simulink library "sadc_library_old"  (R2020b)
settings: Solver=VariableStepAuto  StartTime=0.0  StopTime=10.0  RelTol=1e-3
undefined symbols (not defined in the file): actuators, constants, control, magnitude, orbit, sensors
libraries: vrlib x12
(part 1 of 2)
settings Model: Creator=loren  LastModifiedBy=loren

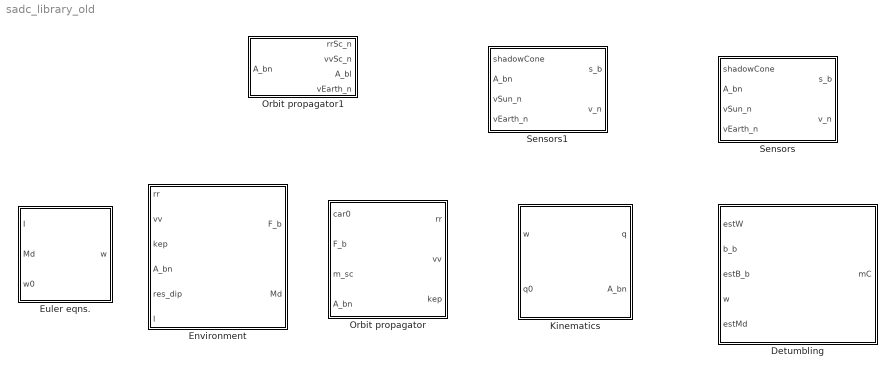
== system sadc_library_old ==
  Detumbling : Subsystem
  Environment : Subsystem
  Euler eqns. : Subsystem
  Kinematics : Subsystem
  Orbit propagator : Subsystem
  Orbit propagator1 : Subsystem
  Sensors : Subsystem
  Sensors1 : Subsystem

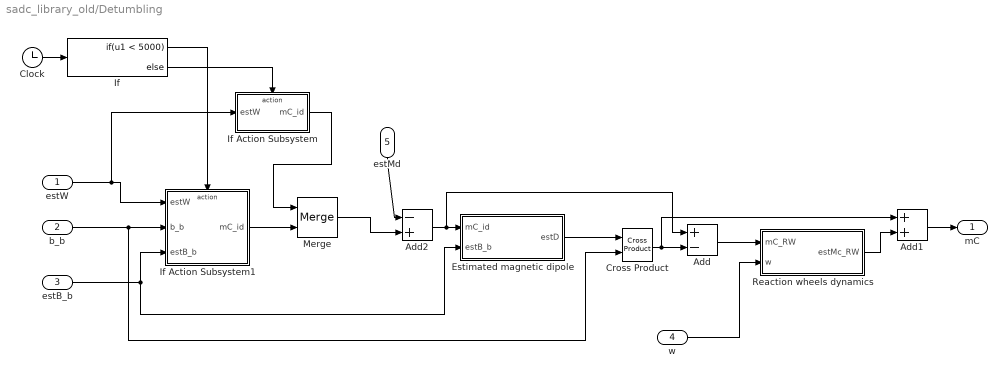
== system sadc_library_old/Detumbling ==
  estW : Inport
  b_b : Inport  Port=2
  estB_b : Inport  Port=3
  w : Inport  Port=4
  estMd : Inport  Port=5
  Add : Sum  Inputs=+-
  Add1 : Sum
  Add2 : Sum  Inputs=-+
  Clock : Clock
  Cross Product : vrlib/Utilities/Cross Product
  Estimated magnetic dipole : Subsystem
  If : If  IfExpression=u1 < 5000
  If Action Subsystem : Subsystem  TreatAsAtomicUnit=on
  If Action Subsystem1 : Subsystem  TreatAsAtomicUnit=on
  Merge : Merge
  Reaction wheels dynamics : Subsystem
  mC : Outport
  wires:
  estW/1 -> If Action Subsystem/1(estW), If Action Subsystem1/1(estW)
  b_b/1 -> If Action Subsystem1/2(b_b), Cross Product/2
  estB_b/1 -> If Action Subsystem1/3(estB_b), Estimated magnetic dipole/2(estB_b)
  If Action Subsystem1/1(mC_id) -> Merge/2
  Estimated magnetic dipole/1(estD) -> Cross Product/1
  Cross Product/1 -> Add1/1, Add/2
  Add/1 -> Reaction wheels dynamics/1(mC_RW)
  w/1 -> Reaction wheels dynamics/2(w)
  Reaction wheels dynamics/1(estMc_RW) -> Add1/2
  Add1/1 -> mC/1
  Add2/1 -> Estimated magnetic dipole/1(mC_id), Add/1
  estMd/1 -> Add2/1
  Clock/1 -> If/1
  Merge/1 -> Add2/2
  If/1 -> If Action Subsystem1/Action
  If/2 -> If Action Subsystem/Action
  If Action Subsystem/1(mC_id) -> Merge/1

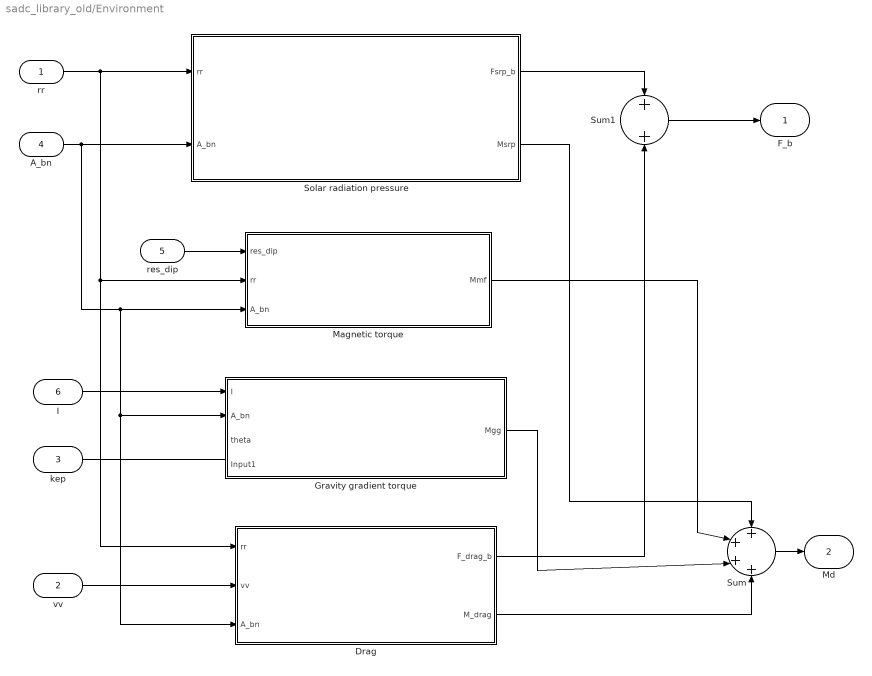
== system sadc_library_old/Environment ==
  rr : Inport
  vv : Inport  Port=2
  kep : Inport  Port=3
  A_bn : Inport  Port=4
  res_dip : Inport  Port=5
  I : Inport  Port=6
  Drag : Subsystem
  Gravity gradient torque : Subsystem
  Magnetic torque : Subsystem
  Solar radiation pressure : Subsystem
  Sum : Sum  Inputs=++++
  Sum1 : Sum
  F_b : Outport
  Md : Outport  Port=2
  wires:
  kep/1 -> ?
  Solar radiation pressure/1(Fsrp_b) -> Sum1/1
  Solar radiation pressure/2(Msrp) -> Sum/1
  A_bn/1 -> Drag/3(A_bn), Gravity gradient torque/2(A_bn), Magnetic torque/3(A_bn), Solar radiation pressure/2(A_bn)
  vv/1 -> Drag/2(vv)
  rr/1 -> Magnetic torque/2(rr), Drag/1(rr), Solar radiation pressure/1(rr)
  Gravity gradient torque/1(Mgg) -> Sum/3
  Drag/2(M_drag) -> Sum/4
  Drag/1(F_drag_b) -> Sum1/2
  I/1 -> Gravity gradient torque/1(I)
  res_dip/1 -> Magnetic torque/1(res_dip)
  Magnetic torque/1(Mmf) -> Sum/2
  Sum1/1 -> F_b/1
  Sum/1 -> Md/1

== system sadc_library_old/Euler eqns. ==
  I : Inport
  Md : Inport  Port=2
  w0 : Inport  Port=3
  Add : Sum  Inputs=-+
  Cross Product : vrlib/Utilities/Cross Product
  Divide : Product  Inputs=/*  Multiplication=Matrix(*)
  Integrator : Integrator  InitialConditionSource=external
  Product : Product  Multiplication=Matrix(*)
  w : Outport
  wires:
  I/1 -> Divide/1, Product/1
  w0/1 -> Integrator/2
  Integrator/1 -> Product/2, w/1, Cross Product/2  "w"
  Product/1 -> Cross Product/1
  Md/1 -> Add/2
  Cross Product/1 -> Add/1
  Add/1 -> Divide/2
  Divide/1 -> Integrator/1

== system sadc_library_old/Kinematics ==
  w : Inport
  q0 : Inport  Port=2
  DCM : Subsystem
  Quaternion integration : Subsystem
  q : Outport
  A_bn : Outport  Port=2
  wires:
  w/1 -> Quaternion integration/1(w)
  q0/1 -> Quaternion integration/2(q0)
  Quaternion integration/1(q) -> q/1, DCM/1(q)
  DCM/1(A_bn) -> A_bn/1

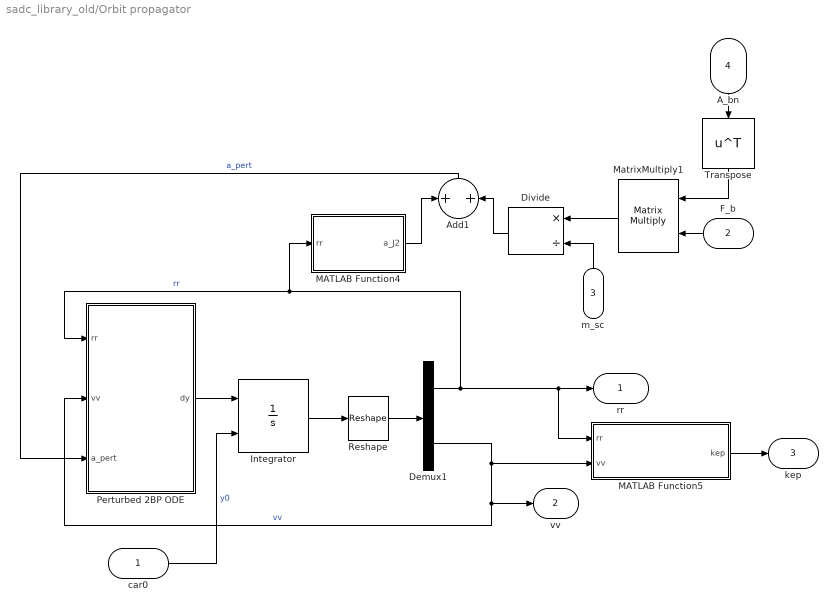
== system sadc_library_old/Orbit propagator ==
  car0 : Inport
  F_b : Inport  Port=2
  m_sc : Inport  Port=3
  A_bn : Inport  Port=4
  Add1 : Sum
  Demux1 : Demux  Outputs=[3,3]
  Divide : Product  Inputs=*/
  Integrator : Integrator  InitialConditionSource=external
  MATLAB Function4 : MATLAB Function  TreatAsAtomicUnit=on
  MATLAB Function5 : MATLAB Function  TreatAsAtomicUnit=on
  MatrixMultiply1 : Product  Multiplication=Matrix(*)
  Perturbed 2BP ODE : Subsystem
  Reshape : Reshape  OutputDimensionality=Column vector (2-D)
  Transpose : Math  Operator=transpose  SaturateOnIntegerOverflow=on
  rr : Outport
  vv : Outport  Port=2
  kep : Outport  Port=3
  wires:
  Integrator/1 -> Reshape/1
  Demux1/1 -> MATLAB Function5/1(rr), rr/1, MATLAB Function4/1(rr), Perturbed 2BP ODE/1(rr)  "rr"
  Perturbed 2BP ODE/1(dy) -> Integrator/1
  Demux1/2 -> vv/1, Perturbed 2BP ODE/2(vv), MATLAB Function5/2(vv)  "vv"
  car0/1 -> Integrator/2  "y0"
  Add1/1 -> Perturbed 2BP ODE/3(a_pert)  "a_pert"
  MATLAB Function4/1(a_J2) -> Add1/1
  F_b/1 -> MatrixMultiply1/2
  MatrixMultiply1/1 -> Divide/1
  m_sc/1 -> Divide/2
  Divide/1 -> Add1/2
  MATLAB Function5/1(kep) -> kep/1
  A_bn/1 -> Transpose/1
  Transpose/1 -> MatrixMultiply1/1
  Reshape/1 -> Demux1/1

== system sadc_library_old/Orbit propagator1 ==
  A_bn : Inport
  Gain : Gain
  Integrator : Integrator  InitialCondition=orbit.theta0
  LVLH frame : Subsystem
  Normalize Vector : vrlib/Utilities/Normalize Vector  maxzero=0
  Position and velocity (inertial frame) : Subsystem
  True anomaly ODE : Subsystem
  rrSc_n : Outport
  vvSc_n : Outport  Port=2
  A_bl : Outport  Port=3
  vEarth_n : Outport  Port=4
  wires:
  Gain/1 -> vEarth_n/1
  Normalize Vector/1 -> Gain/1
  A_bn/1 -> LVLH frame/2(A_bn)
  LVLH frame/1(A_bl) -> A_bl/1
  Position and velocity (inertial frame)/2(vvSc_n) -> vvSc_n/1
  Position and velocity (inertial frame)/1(rrSc_n) -> rrSc_n/1, Normalize Vector/1
  Integrator/1 -> LVLH frame/1(theta), Position and velocity (inertial frame)/1(theta), True anomaly ODE/1(theta)
  True anomaly ODE/1(theta_dot) -> Integrator/1

== system sadc_library_old/Sensors ==
  shadowCone : Inport
  A_bn : Inport  Port=2
  vSun_n : Inport  Port=3
  vEarth_n : Inport  Port=4
  Eclipse (S.T + E.H sensors) : Subsystem  TreatAsAtomicUnit=on
  Merge : Merge
  Merge2 : Merge
  Sunlight (S.S + E.H sensors) : Subsystem  TreatAsAtomicUnit=on
  s_b : Outport
  v_n : Outport  Port=2
  wires:
  shadowCone/1 -> Eclipse (S.T + E.H sensors)/Enable, Sunlight (S.S + E.H sensors)/Enable
  A_bn/1 -> Eclipse (S.T + E.H sensors)/1(A_bn), Sunlight (S.S + E.H sensors)/1(A_bn)
  vSun_n/1 -> Sunlight (S.S + E.H sensors)/2(vSun_n)
  vEarth_n/1 -> Sunlight (S.S + E.H sensors)/3(vEarth_n), Eclipse (S.T + E.H sensors)/2(vEarth_n)
  Merge/1 -> s_b/1
  Merge2/1 -> v_n/1
  Eclipse (S.T + E.H sensors)/1(s_b) -> Merge/1
  Sunlight (S.S + E.H sensors)/1(s_b) -> Merge/2
  Sunlight (S.S + E.H sensors)/2(v_n) -> Merge2/2
  Eclipse (S.T + E.H sensors)/2(v_n) -> Merge2/1

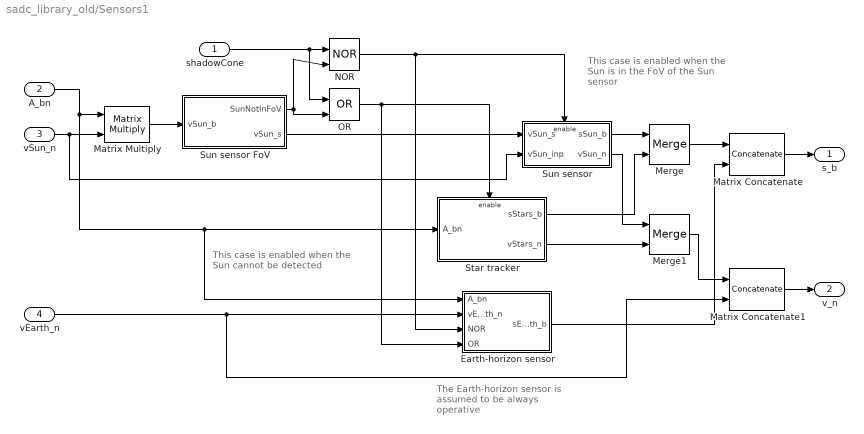
== system sadc_library_old/Sensors1 ==
  note: The Earth-horizon sensor
      | is assumed to be always
      | operative
  note: This case is enabled when
      | the Sun cannot be detected
  note: This case is enabled when
      | the Sun is in the FoV
      | of the Sun sensor
  shadowCone : Inport
  A_bn : Inport  Port=2
  vSun_n : Inport  Port=3
  vEarth_n : Inport  Port=4
  Earth-horizon sensor : Subsystem
  Matrix Concatenate : Concatenate  Mode=Multidimensional array  ConcatenateDimension=2
  Matrix Concatenate1 : Concatenate  Mode=Multidimensional array  ConcatenateDimension=2
  Matrix Multiply : Product  Multiplication=Matrix(*)
  Merge : Merge
  Merge1 : Merge
  NOR : Logic  Operator=NOR  IconShape=distinctive  AllPortsSameDT=off  OutDataTypeStr=boolean
  OR : Logic  Operator=OR  IconShape=distinctive  AllPortsSameDT=off  OutDataTypeStr=boolean
  Star tracker : Subsystem
  Sun sensor : Subsystem
  Sun sensor FoV : Subsystem
  s_b : Outport
  v_n : Outport  Port=2
  wires:
  A_bn/1 -> Earth-horizon sensor/1(A_bn), Star tracker/1(A_bn), Matrix Multiply/1
  vSun_n/1 -> Sun sensor/2(vSun_inp), Matrix Multiply/2
  Matrix Multiply/1 -> Sun sensor FoV/1(vSun_b)
  shadowCone/1 -> NOR/1, OR/1
  Sun sensor FoV/1(SunNotInFoV) -> NOR/2, OR/2
  Sun sensor FoV/2(vSun_s) -> Sun sensor/1(vSun_s)
  OR/1 -> Star tracker/Enable, Earth-horizon sensor/4(OR)
  vEarth_n/1 -> Matrix Concatenate1/2, Earth-horizon sensor/2(vEarth_n)
  Sun sensor/1(sSun_b) -> Merge/1
  Star tracker/1(sStars_b) -> Merge/2
  Star tracker/2(vStars_n) -> Merge1/2
  Matrix Concatenate1/1 -> v_n/1
  Matrix Concatenate/1 -> s_b/1
  Sun sensor/2(vSun_n) -> Merge1/1
  Merge/1 -> Matrix Concatenate/1
  Earth-horizon sensor/1(sEarth_b) -> Matrix Concatenate/2
  Merge1/1 -> Matrix Concatenate1/1
  NOR/1 -> Sun sensor/Enable, Earth-horizon sensor/3(NOR)

== system sadc_library_old/Detumbling/Estimated magnetic dipole ==
  mC_id : Inport
  estB_b : Inport  Port=2
  Cross Product : vrlib/Utilities/Cross Product
  Divide : Product  Inputs=/*
  Dot Product : DotProduct  InputSameDT=on  OutDataTypeStr=Inherit: Inherit via internal rule
  Saturation : Saturate  UpperLimit=actuators.mt.D_max  LowerLimit=actuators.mt.D_min
  estD : Outport
  wires:
  Divide/1 -> Saturation/1
  Dot Product/1 -> Divide/1
  Cross Product/1 -> Divide/2
  estB_b/1 -> Dot Product/1, Dot Product/2, Cross Product/1
  mC_id/1 -> Cross Product/2
  Saturation/1 -> estD/1

== system sadc_library_old/Detumbling/If Action Subsystem ==
  estW : Inport
  Action Port : ActionPort
  Gain : Gain  Gain=-control.detumbling.kp
  mC_id : Outport
  wires:
  estW/1 -> Gain/1
  Gain/1 -> mC_id/1

== system sadc_library_old/Detumbling/If Action Subsystem1 ==
  estW : Inport
  b_b : Inport  Port=2
  estB_b : Inport  Port=3
  Action Port : ActionPort
  Cross Product : vrlib/Utilities/Cross Product
  Cross Product1 : vrlib/Utilities/Cross Product
  Gain : Gain  Gain=-control.detumbling.kb
  mC_id : Outport
  wires:
  Cross Product1/1 -> mC_id/1
  estB_b/1 -> Cross Product/1
  estW/1 -> Cross Product/2
  b_b/1 -> Cross Product1/2
  Gain/1 -> Cross Product1/1
  Cross Product/1 -> Gain/1

== system sadc_library_old/Detumbling/Reaction wheels dynamics ==
  mC_RW : Inport
  w : Inport  Port=2
  Add : Sum
  Add1 : Sum  Inputs=--
  Cross Product : vrlib/Utilities/Cross Product
  Gain : Gain  Gain=actuators.rw.A  Multiplication=Matrix(K*u) (u vector)
  Gain1 : Gain  Gain=-actuators.rw.A_star  Multiplication=Matrix(K*u) (u vector)
  Gain2 : Gain  Gain=actuators.rw.A  Multiplication=Matrix(K*u) (u vector)
  Integrator : Integrator  InitialCondition=[0;0;0;0]
  Saturation : Saturate  UpperLimit=actuators.rw.h_max  LowerLimit=-actuators.rw.h_max
  estMc_RW : Outport
  wires:
  mC_RW/1 -> Add/1
  w/1 -> Cross Product/1
  Gain/1 -> Cross Product/2
  Cross Product/1 -> Add1/1, Add/2
  Gain1/1 -> Integrator/1, Gain2/1  "hr_dot"
  Integrator/1 -> Saturation/1  "h_r"
  Saturation/1 -> Gain/1
  Gain2/1 -> Add1/2
  Add1/1 -> estMc_RW/1
  Add/1 -> Gain1/1

== system sadc_library_old/Environment/Drag ==
  rr : Inport
  vv : Inport  Port=2
  A_bn : Inport  Port=3
  Density @ 400 km : Constant  Value=3.725*1e-12
  MATLAB Function1 : MATLAB Function  TreatAsAtomicUnit=on
  F_drag_b : Outport
  M_drag : Outport  Port=2
  wires:
  rr/1 -> MATLAB Function1/1(rr)
  MATLAB Function1/1(Fdrag_b) -> F_drag_b/1
  MATLAB Function1/2(Mdrag) -> M_drag/1
  vv/1 -> MATLAB Function1/2(vv)
  A_bn/1 -> MATLAB Function1/3(A_bn)
  Density @ 400 km/1 -> MATLAB Function1/4(rho)

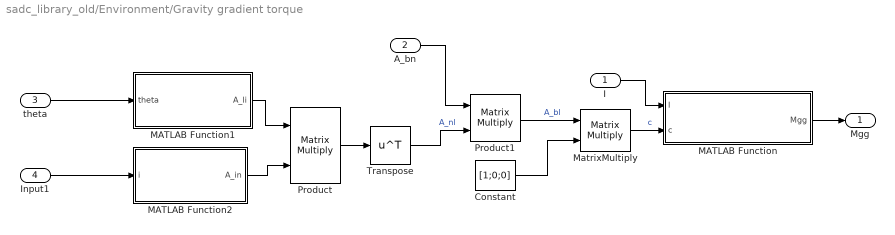
== system sadc_library_old/Environment/Gravity gradient torque ==
  I : Inport
  A_bn : Inport  Port=2
  theta : Inport  Port=3
  Input1 : Inport  Port=4
  Constant : Constant  Value=[1;0;0]
  MATLAB Function : MATLAB Function  TreatAsAtomicUnit=on
  MATLAB Function1 : MATLAB Function  TreatAsAtomicUnit=on
  MATLAB Function2 : MATLAB Function  TreatAsAtomicUnit=on
  MatrixMultiply : Product  Multiplication=Matrix(*)
  Product : Product  Multiplication=Matrix(*)
  Product1 : Product  Multiplication=Matrix(*)
  Transpose : Math  Operator=transpose  SaturateOnIntegerOverflow=on
  Mgg : Outport
  wires:
  I/1 -> MATLAB Function/1(I)
  Product/1 -> Transpose/1
  Transpose/1 -> Product1/2  "A_nl"
  Product1/1 -> MatrixMultiply/1  "A_bl"
  A_bn/1 -> Product1/1
  Constant/1 -> MatrixMultiply/2
  MatrixMultiply/1 -> MATLAB Function/2(c)  "c"
  MATLAB Function/1(Mgg) -> Mgg/1
  MATLAB Function2/1(A_in) -> Product/2
  MATLAB Function1/1(A_li) -> Product/1
  theta/1 -> MATLAB Function1/1(theta)
  Input1/1 -> MATLAB Function2/1(i)

== system sadc_library_old/Environment/Magnetic torque ==
  res_dip : Inport
  rr : Inport  Port=2
  A_bn : Inport  Port=3
  Clock : Clock
  Cross Product : vrlib/Utilities/Cross Product
  MATLAB Function : MATLAB Function  TreatAsAtomicUnit=on
  MATLAB Function1 : MATLAB Function  TreatAsAtomicUnit=on
  Mmf : Outport
  wires:
  Cross Product/1 -> Mmf/1
  Clock/1 -> MATLAB Function1/1(t)
  rr/1 -> MATLAB Function/2(rr)
  A_bn/1 -> MATLAB Function/3(A_bn)
  res_dip/1 -> Cross Product/1
  MATLAB Function/1(b_b) -> Cross Product/2
  MATLAB Function1/1(m) -> MATLAB Function/1(m)

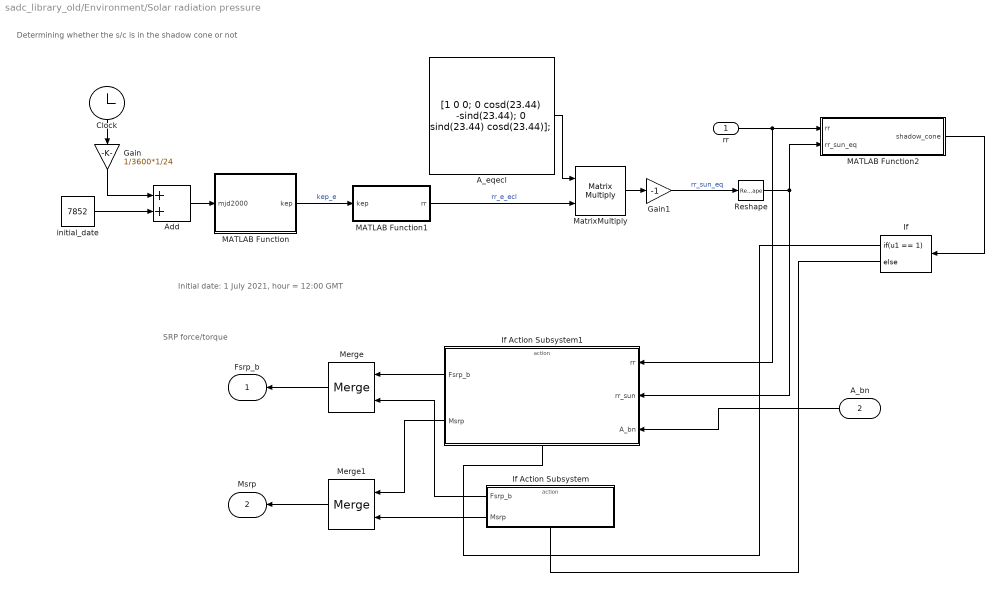
== system sadc_library_old/Environment/Solar radiation pressure ==
  note: SRP force/torque
  note: Initial date: 1 July 2021,
      | hour = 12:00 GMT
  note: Determining whether the s/c is in the shadow cone or not
  rr : Inport
  A_bn : Inport  Port=2
  A_eqecl : Constant  Value=|
      | [1   0   0;
      |     0  cosd(23.44)  -sind(23.44);
      |     0  sind(23.44)  cosd(23.44)];
  Add : Sum
  Clock : Clock
  Gain : Gain  Gain=1/3600*1/24
  Gain1 : Gain  Gain=-1
  If : If  IfExpression=u1 == 1
  If Action Subsystem : Subsystem  TreatAsAtomicUnit=on
  If Action Subsystem1 : Subsystem  TreatAsAtomicUnit=on
  MATLAB Function : MATLAB Function  TreatAsAtomicUnit=on
  MATLAB Function1 : MATLAB Function  TreatAsAtomicUnit=on
  MATLAB Function2 : MATLAB Function  TreatAsAtomicUnit=on
  MatrixMultiply : Product  Multiplication=Matrix(*)
  Merge : Merge
  Merge1 : Merge
  Reshape : Reshape  OutputDimensionality=Column vector (2-D)
  initial_date : Constant  Value=7852
  Fsrp_b : Outport
  Msrp : Outport  Port=2
  wires:
  initial_date/1 -> Add/2
  Clock/1 -> Gain/1
  Add/1 -> MATLAB Function/1(mjd2000)
  Gain/1 -> Add/1
  MatrixMultiply/1 -> Gain1/1
  MATLAB Function1/1(rr) -> MatrixMultiply/2  "rr_e_ecl"
  MATLAB Function/1(kep) -> MATLAB Function1/1(kep)  "kep_e"
  Gain1/1 -> Reshape/1  "rr_sun_eq"
  MATLAB Function2/1(shadow_cone) -> If/1
  If/2 -> If Action Subsystem/Action
  If/1 -> If Action Subsystem1/Action
  If Action Subsystem/1(Fsrp_b) -> Merge/2
  If Action Subsystem/2(Msrp) -> Merge1/2
  rr/1 -> MATLAB Function2/1(rr), If Action Subsystem1/1(rr)
  Merge/1 -> Fsrp_b/1
  Merge1/1 -> Msrp/1
  If Action Subsystem1/1(Fsrp_b) -> Merge/1
  If Action Subsystem1/2(Msrp) -> Merge1/1
  A_bn/1 -> If Action Subsystem1/3(A_bn)
  A_eqecl/1 -> MatrixMultiply/1
  Reshape/1 -> MATLAB Function2/2(rr_sun_eq), If Action Subsystem1/2(rr_sun)

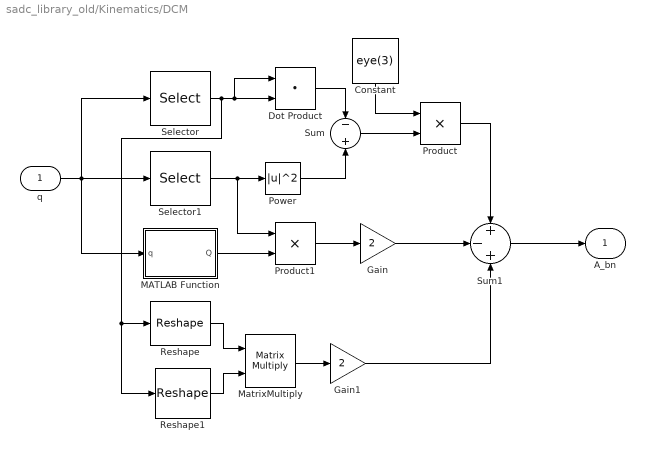
== system sadc_library_old/Kinematics/DCM ==
  q : Inport
  Constant : Constant  Value=eye(3)
  Dot Product : DotProduct  InputSameDT=on  OutDataTypeStr=Inherit: Inherit via internal rule
  Gain : Gain  Gain=2
  Gain1 : Gain  Gain=2
  MATLAB Function : MATLAB Function  TreatAsAtomicUnit=on
  MatrixMultiply : Product  Multiplication=Matrix(*)
  Power : Math  Operator=magnitude^2  SaturateOnIntegerOverflow=on
  Product : Product
  Product1 : Product
  Reshape : Reshape  OutputDimensionality=Column vector (2-D)
  Reshape1 : Reshape  OutputDimensionality=Row vector (2-D)
  Selector : Selector  InputPortWidth=4  IndexOptions=Index vector (dialog)  Indices=[1 2 3]  OutputSizes=1
  Selector1 : Selector  InputPortWidth=4  IndexOptions=Index vector (dialog)  Indices=[4]  OutputSizes=1
  Sum : Sum  Inputs=-+
  Sum1 : Sum  Inputs=+-+
  A_bn : Outport
  wires:
  q/1 -> MATLAB Function/1(q), Selector1/1, Selector/1
  Selector/1 -> Reshape1/1, Reshape/1, Dot Product/2, Dot Product/1
  Selector1/1 -> Product1/1, Power/1
  Power/1 -> Sum/2
  Dot Product/1 -> Sum/1
  Constant/1 -> Product/1
  Sum/1 -> Product/2
  MATLAB Function/1(Q) -> Product1/2
  Product1/1 -> Gain/1
  Reshape/1 -> MatrixMultiply/1
  Reshape1/1 -> MatrixMultiply/2
  MatrixMultiply/1 -> Gain1/1
  Product/1 -> Sum1/1
  Gain/1 -> Sum1/2
  Gain1/1 -> Sum1/3
  Sum1/1 -> A_bn/1

== system sadc_library_old/Kinematics/Quaternion integration ==
  w : Inport
  q0 : Inport  Port=2
  Gain : Gain  Gain=1/2
  Integrator : Integrator  InitialConditionSource=external
  MATLAB Function : MATLAB Function  TreatAsAtomicUnit=on
  MatrixMultiply : Product  Multiplication=Matrix(*)
  Normalize Vector : vrlib/Utilities/Normalize Vector  maxzero=0
  q : Outport
  wires:
  Integrator/1 -> Normalize Vector/1
  w/1 -> MATLAB Function/1(w)
  Normalize Vector/1 -> q/1, MatrixMultiply/2
  q0/1 -> Integrator/2
  MATLAB Function/1(OM_mat) -> MatrixMultiply/1
  MatrixMultiply/1 -> Gain/1
  Gain/1 -> Integrator/1

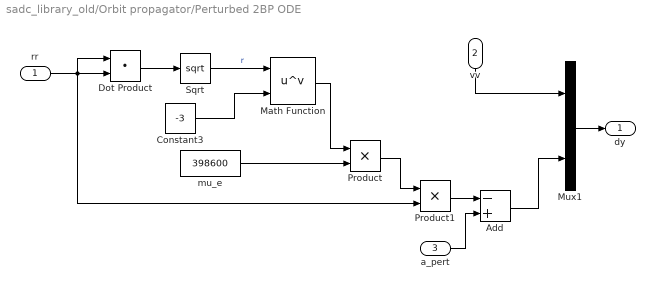
== system sadc_library_old/Orbit propagator/Perturbed 2BP ODE ==
  rr : Inport
  vv : Inport  Port=2
  a_pert : Inport  Port=3
  Add : Sum  Inputs=-+
  Constant3 : Constant  Value=-3
  Dot Product : DotProduct  InputSameDT=on  OutDataTypeStr=Inherit: Inherit via internal rule
  Math Function : Math  Operator=pow  SaturateOnIntegerOverflow=on
  Mux1 : Mux  Inputs=[3,3]
  Product : Product
  Product1 : Product
  Sqrt : Sqrt  SaturateOnIntegerOverflow=on
  mu_e : Constant  Value=398600
  dy : Outport
  wires:
  rr/1 -> Dot Product/1, Product1/2, Dot Product/2
  Add/1 -> Mux1/2
  Math Function/1 -> Product/1
  Mux1/1 -> dy/1
  Dot Product/1 -> Sqrt/1
  Product1/1 -> Add/1
  Product/1 -> Product1/1
  Constant3/1 -> Math Function/2
  a_pert/1 -> Add/2
  Sqrt/1 -> Math Function/1  "r"
  vv/1 -> Mux1/1
  mu_e/1 -> Product/2

== system sadc_library_old/Orbit propagator1/LVLH frame ==
  theta : Inport
  A_bn : Inport  Port=2
  LVLH to inclined orbit frame : Subsystem
  Product : Product  Multiplication=Matrix(*)
  Product1 : Product  Multiplication=Matrix(*)
  R1(i) : Constant  Value=[1 0 0; 0 cos(orbit.i) sin(orbit.i); 0 -sin(orbit.i) cos(orbit.i)];
  Transpose : Math  Operator=transpose  SaturateOnIntegerOverflow=on
  A_bl : Outport
  wires:
  LVLH to inclined orbit frame/1(A_li) -> Product/1
  theta/1 -> LVLH to inclined orbit frame/1(theta)
  R1(i)/1 -> Product/2
  Product1/1 -> A_bl/1  "A_bl"
  A_bn/1 -> Product1/1
  Product/1 -> Transpose/1
  Transpose/1 -> Product1/2  "A_nl"

== system sadc_library_old/Orbit propagator1/Position and velocity (inertial frame) ==
  theta : Inport
  MatrixMultiply : Product  Multiplication=Matrix(*)
  MatrixMultiply1 : Product  Multiplication=Matrix(*)
  Position and velocity (perifocal frame) : Subsystem
  R1(i) : Constant  Value=[1 0 0; 0 cos(orbit.i) sin(orbit.i); 0 -sin(orbit.i) cos(orbit.i)];
  R3(OM) : Constant  Value=[cos(orbit.OM), sin(orbit.OM), 0; -sin(orbit.OM), cos(orbit.OM), 0; 0, 0, 1]
  R3(om) : Constant  Value=[cos(orbit.om), sin(orbit.om), 0; -sin(orbit.om), cos(orbit.om), 0; 0, 0, 1]
  Rotation matrix (perifocal-inertial) : Product  Inputs=3  Multiplication=Matrix(*)
  Transpose : Math  Operator=transpose  SaturateOnIntegerOverflow=on
  rrSc_n : Outport
  vvSc_n : Outport  Port=2
  wires:
  theta/1 -> Position and velocity (perifocal frame)/1(theta)
  Position and velocity (perifocal frame)/1(rrSc_pf) -> MatrixMultiply/2
  R3(OM)/1 -> Rotation matrix (perifocal-inertial)/3
  Transpose/1 -> MatrixMultiply/1, MatrixMultiply1/1
  Rotation matrix (perifocal-inertial)/1 -> Transpose/1
  R1(i)/1 -> Rotation matrix (perifocal-inertial)/2
  R3(om)/1 -> Rotation matrix (perifocal-inertial)/1
  MatrixMultiply1/1 -> vvSc_n/1
  Position and velocity (perifocal frame)/2(vvSc_pf) -> MatrixMultiply1/2
  MatrixMultiply/1 -> rrSc_n/1

== system sadc_library_old/Orbit propagator1/True anomaly ODE ==
  theta : Inport
  Add : Sum
  Constant1 : Constant
  Cos : Trigonometry  Operator=cos
  Gain : Gain  Gain=sqrt(constants.mu/orbit.a^3)
  Gain1 : Gain  Gain=(1 - orbit.e^2)^(-3/2)
  Gain2 : Gain  Gain=orbit.e
  Power : Math  Operator=square  SaturateOnIntegerOverflow=on
  theta_dot : Outport
  wires:
  Gain1/1 -> theta_dot/1
  Gain/1 -> Gain1/1
  Power/1 -> Gain/1
  Add/1 -> Power/1
  Gain2/1 -> Add/2
  Cos/1 -> Gain2/1
  Constant1/1 -> Add/1
  theta/1 -> Cos/1

== system sadc_library_old/Sensors/Eclipse (S.T + E.H sensors) ==
  A_bn : Inport
  vEarth_n : Inport  Port=2
  Enable : EnablePort
  Earth-horizon sensor : Subsystem  AncestorBlock=|
      | library/Sensors/Sunlight
      | (S.S + E.H sensors)/Earth-horizon sensor
  Star tracker : Subsystem
  Vector Concatenate : Concatenate  Mode=Multidimensional array  ConcatenateDimension=2
  Vector Concatenate1 : Concatenate  Mode=Multidimensional array  ConcatenateDimension=2
  s_b : Outport
  v_n : Outport  Port=2
  wires:
  Vector Concatenate1/1 -> v_n/1
  Vector Concatenate/1 -> s_b/1
  Earth-horizon sensor/1(vEarth_b) -> Vector Concatenate/1
  A_bn/1 -> Star tracker/1(A_bn), Earth-horizon sensor/1(A_bn)
  vEarth_n/1 -> Vector Concatenate1/1, Earth-horizon sensor/2(vEarth_n)
  Star tracker/1(sStars_b) -> Vector Concatenate/2
  Star tracker/2(vStars_n) -> Vector Concatenate1/2

== system sadc_library_old/Sensors/Sunlight (S.S + E.H sensors) ==
  A_bn : Inport
  vSun_n : Inport  Port=2
  vEarth_n : Inport  Port=3
  Enable : EnablePort
  Earth-horizon sensor : Subsystem
  Sun sensor : Subsystem
  Vector Concatenate : Concatenate  Mode=Multidimensional array  ConcatenateDimension=2
  Vector Concatenate1 : Concatenate  Mode=Multidimensional array  ConcatenateDimension=2
  s_b : Outport
  v_n : Outport  Port=2
  wires:
  A_bn/1 -> Sun sensor/1(A_bn), Earth-horizon sensor/1(A_bn)
  vSun_n/1 -> Sun sensor/2(vSun_n), Vector Concatenate1/1
  vEarth_n/1 -> Vector Concatenate1/2, Earth-horizon sensor/2(vEarth_n)
  Sun sensor/1(vSun_b) -> Vector Concatenate/1
  Earth-horizon sensor/1(vEarth_b) -> Vector Concatenate/2
  Vector Concatenate/1 -> s_b/1
  Vector Concatenate1/1 -> v_n/1

== system sadc_library_old/Sensors1/Earth-horizon sensor ==
  A_bn : Inport
  vEarth_n : Inport  Port=2
  NOR : Inport  Port=3
  OR : Inport  Port=4
  Constant : Constant  Value=sensors.eh.A_sb
  Determination of the sampling time : Subsystem
  MATLAB Function : MATLAB Function  TreatAsAtomicUnit=on
  MatrixMultiply : Product  Multiplication=Matrix(*)
  MatrixMultiply1 : Product  Multiplication=Matrix(*)
  MatrixMultiply2 : Product  Multiplication=Matrix(*)
  Zero-Order Hold : ZeroOrderHold  SampleTime=max([sensors.ss.Ts, sensors.eh.Ts])
  sEarth_b : Outport
  wires:
  Zero-Order Hold/1 -> MatrixMultiply1/2
  vEarth_n/1 -> MatrixMultiply2/2
  MATLAB Function/1(A_err) -> MatrixMultiply1/1
  A_bn/1 -> MatrixMultiply2/1
  MatrixMultiply1/1 -> sEarth_b/1
  MatrixMultiply/1 -> Zero-Order Hold/1  "vEarth_s"
  MatrixMultiply2/1 -> MatrixMultiply/2
  Constant/1 -> MatrixMultiply/1
  Determination of the sampling time/1(phi) -> MATLAB Function/1(phi)
  Determination of the sampling time/2(theta) -> MATLAB Function/2(theta)
  Determination of the sampling time/3(psi) -> MATLAB Function/3(psi)
  NOR/1 -> Determination of the sampling time/1(NOR)
  OR/1 -> Determination of the sampling time/2(OR)

== system sadc_library_old/Sensors1/Star tracker ==
  A_bn : Inport
  Enable : EnablePort
  MATLAB Function : MATLAB Function  TreatAsAtomicUnit=on
  Memory : Memory  InitialCondition=sensors.st.vStars_n_init  InheritSampleTime=on
  Random Number : RandomNumber  Variance=sensors.st.sigmaPhi^2  Seed=randi(1e5,1,1)  SampleTime=max([sensors.eh.Ts, sensors.st.Ts])
  Random Number1 : RandomNumber  Variance=sensors.st.sigmaTheta^2  Seed=randi(1e5,1,1)  SampleTime=max([sensors.eh.Ts, sensors.st.Ts])
  Random Number2 : RandomNumber  Variance=sensors.st.sigmaPsi^2  Seed=randi(1e5,1,1)  SampleTime=max([sensors.eh.Ts, sensors.st.Ts])
  Reshape : Reshape  OutputDimensionality=Customize  OutputDimensions=[sensors.st.nStars*3, 1]
  Reshape1 : Reshape  OutputDimensionality=Customize  OutputDimensions=[sensors.st.nStars*3, 1]
  Zero-Order Hold : ZeroOrderHold  SampleTime=max([sensors.eh.Ts, sensors.st.Ts])
  sStars_b : Outport
  vStars_n : Outport  Port=2
  wires:
  Memory/1 -> MATLAB Function/5(v_n_old)
  MATLAB Function/2(v_n) -> Reshape1/1, Memory/1
  MATLAB Function/1(s_b) -> Reshape/1
  Zero-Order Hold/1 -> MATLAB Function/1(A_bn)
  Random Number/1 -> MATLAB Function/2(phi)
  Random Number2/1 -> MATLAB Function/4(psi)
  A_bn/1 -> Zero-Order Hold/1
  Random Number1/1 -> MATLAB Function/3(theta)
  Reshape/1 -> sStars_b/1
  Reshape1/1 -> vStars_n/1

== system sadc_library_old/Sensors1/Sun sensor ==
  vSun_s : Inport
  vSun_inp : Inport  Port=2
  Enable : EnablePort
  MATLAB Function : MATLAB Function  TreatAsAtomicUnit=on
  MatrixMultiply1 : Product  Multiplication=Matrix(*)
  Random Number : RandomNumber  Variance=sensors.ss.sigmaPhi^2  Seed=randi(1e5, 1, 1)  SampleTime=max([sensors.ss.Ts, sensors.eh.Ts])
  Random Number1 : RandomNumber  Variance=sensors.ss.sigmaTheta^2  Seed=randi(1e5, 1, 1)  SampleTime=max([sensors.ss.Ts, sensors.eh.Ts])
  Random Number2 : RandomNumber  Variance=sensors.ss.sigmaPsi^2  Seed=randi(1e5, 1, 1)  SampleTime=max([sensors.ss.Ts, sensors.eh.Ts])
  Zero-Order Hold : ZeroOrderHold  SampleTime=max([sensors.ss.Ts, sensors.eh.Ts])
  sSun_b : Outport
  vSun_n : Outport  Port=2
  wires:
  Zero-Order Hold/1 -> MatrixMultiply1/2
  vSun_s/1 -> Zero-Order Hold/1  "vSun_s"
  Random Number2/1 -> MATLAB Function/3(psi)
  MatrixMultiply1/1 -> sSun_b/1
  MATLAB Function/1(A_err) -> MatrixMultiply1/1
  Random Number1/1 -> MATLAB Function/2(theta)
  Random Number/1 -> MATLAB Function/1(phi)
  vSun_inp/1 -> vSun_n/1

== system sadc_library_old/Sensors1/Sun sensor FoV ==
  vSun_b : Inport
  Acos : Trigonometry  Operator=acos
  Constant : Constant  Value=sensors.ss.FoV/2
  Constant1 : Constant  Value=sensors.ss.A_sb
  Dot Product : DotProduct  InputSameDT=on  OutDataTypeStr=Inherit: Inherit via internal rule
  Gain : Gain  Gain=sensors.ss.A_sb  Multiplication=Matrix(K*u) (u vector)
  Less Than : RelationalOperator  Operator=>  OutDataTypeStr=boolean  RndMeth=Simplest
  Normalize Vector : vrlib/Utilities/Normalize Vector  maxzero=0
  Selector : Selector  NumberOfDimensions=2  InputPortWidth=3  IndexOptions=Index vector (dialog),Index vector (dialog)  Indices=[1 2 3],[1]  OutputSizes=1,1
  SunNotInFoV : Outport
  vSun_s : Outport  Port=2
  wires:
  Gain/1 -> vSun_s/1, Dot Product/2
  Selector/1 -> Normalize Vector/1
  Normalize Vector/1 -> Dot Product/1
  vSun_b/1 -> Gain/1
  Dot Product/1 -> Acos/1
  Acos/1 -> Less Than/1
  Constant/1 -> Less Than/2
  Less Than/1 -> SunNotInFoV/1
  Constant1/1 -> Selector/1

== system sadc_library_old/Environment/Solar radiation pressure/If Action Subsystem ==
  Action Port : ActionPort
  Constant : Constant  Value=[0;0;0]
  Constant1 : Constant  Value=[0;0;0]
  Fsrp_b : Outport
  Msrp : Outport  Port=2
  wires:
  Constant/1 -> Fsrp_b/1
  Constant1/1 -> Msrp/1

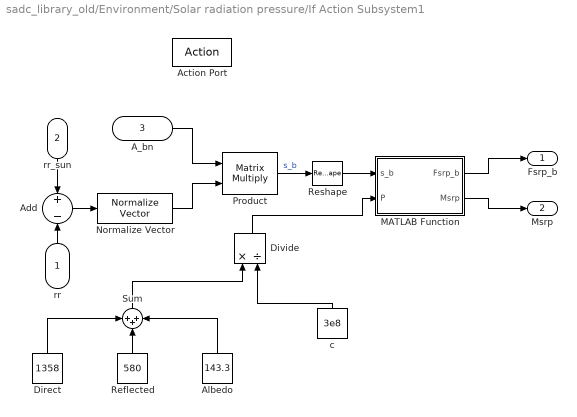
== system sadc_library_old/Environment/Solar radiation pressure/If Action Subsystem1 ==
  rr : Inport
  rr_sun : Inport  Port=2
  A_bn : Inport  Port=3
  Action Port : ActionPort
  Add : Sum  Inputs=+-
  Albedo : Constant  Value=143.3
  Direct : Constant  Value=1358
  Divide : Product  Inputs=*/
  MATLAB Function : MATLAB Function  TreatAsAtomicUnit=on
  Normalize Vector : vrlib/Utilities/Normalize Vector  maxzero=0
  Product : Product  Multiplication=Matrix(*)
  Reflected : Constant  Value=580
  Reshape : Reshape  OutputDimensionality=Column vector (2-D)
  Sum : Sum  Inputs=+++
  c : Constant  Value=3e8
  Fsrp_b : Outport
  Msrp : Outport  Port=2
  wires:
  A_bn/1 -> Product/1
  rr_sun/1 -> Add/1
  Product/1 -> Reshape/1  "s_b"
  Normalize Vector/1 -> Product/2
  Add/1 -> Normalize Vector/1
  MATLAB Function/1(Fsrp_b) -> Fsrp_b/1
  MATLAB Function/2(Msrp) -> Msrp/1
  Reflected/1 -> Sum/2
  Albedo/1 -> Sum/3
  Direct/1 -> Sum/1
  Sum/1 -> Divide/1
  c/1 -> Divide/2
  Divide/1 -> MATLAB Function/2(P)
  rr/1 -> Add/2
  Reshape/1 -> MATLAB Function/1(s_b)

== system sadc_library_old/Orbit propagator1/LVLH frame/LVLH to inclined orbit frame ==
  theta : Inport
  Constant : Constant  Value=0
  Constant1 : Constant  Value=[0 0 1]
  Cos : Trigonometry  Operator=cos
  Gain : Gain  Gain=-1
  Mux : Mux  Inputs=3
  Mux1 : Mux  Inputs=3
  Sin : Trigonometry
  Vector Concatenate : Concatenate  NumInputs=3  Mode=Multidimensional array  ConcatenateDimension=2
  A_li : Outport
  wires:
  Vector Concatenate/1 -> A_li/1
  Mux1/1 -> Vector Concatenate/2
  Constant1/1 -> Vector Concatenate/3
  Mux/1 -> Vector Concatenate/1
  Gain/1 -> Mux1/1
  Constant/1 -> Mux/3, Mux1/3
  Sin/1 -> Mux/2, Gain/1
  Cos/1 -> Mux/1, Mux1/2
  theta/1 -> Cos/1, Sin/1

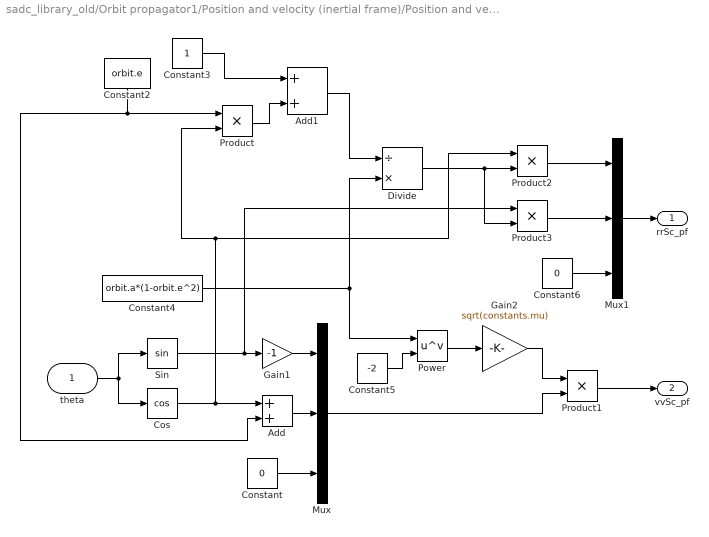
== system sadc_library_old/Orbit propagator1/Position and velocity (inertial frame)/Position and velocity (perifocal frame) ==
  theta : Inport
  Add : Sum
  Add1 : Sum
  Constant : Constant  Value=0
  Constant2 : Constant  Value=orbit.e
  Constant3 : Constant
  Constant4 : Constant  Value=orbit.a*(1-orbit.e^2)
  Constant5 : Constant  Value=-2
  Constant6 : Constant  Value=0
  Cos : Trigonometry  Operator=cos
  Divide : Product  Inputs=/*
  Gain1 : Gain  Gain=-1
  Gain2 : Gain  Gain=sqrt(constants.mu)
  Mux : Mux  Inputs=3
  Mux1 : Mux  Inputs=3
  Power : Math  Operator=pow  SaturateOnIntegerOverflow=on
  Product{,1..3} (4 alike) : Product
  Sin : Trigonometry
  rrSc_pf : Outport
  vvSc_pf : Outport  Port=2
  wires:
  Mux1/1 -> rrSc_pf/1
  Constant6/1 -> Mux1/3
  Product3/1 -> Mux1/2
  Product2/1 -> Mux1/1
  Divide/1 -> Product2/2, Product3/2
  Gain2/1 -> Product1/1
  Power/1 -> Gain2/1
  Constant5/1 -> Power/2
  Constant4/1 -> Power/1, Divide/2
  Add1/1 -> Divide/1
  Product/1 -> Add1/2
  Constant2/1 -> Product/1, Add/2
  Constant3/1 -> Add1/1
  Product1/1 -> vvSc_pf/1
  Constant/1 -> Mux/3
  Add/1 -> Mux/2
  Gain1/1 -> Mux/1
  Cos/1 -> Add/1, Product/2, Product2/1
  Sin/1 -> Gain1/1, Product3/1
  Mux/1 -> Product1/2
  theta/1 -> Sin/1, Cos/1

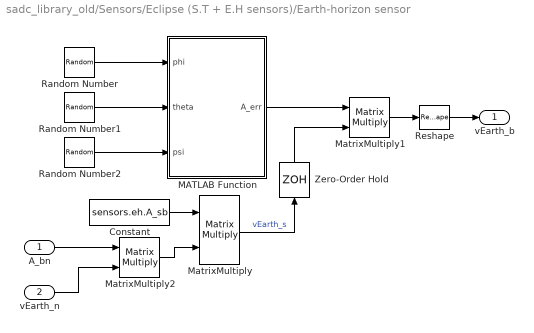
== system sadc_library_old/Sensors/Eclipse (S.T + E.H sensors)/Earth-horizon sensor ==
  A_bn : Inport
  vEarth_n : Inport  Port=2
  Constant : Constant  Value=sensors.eh.A_sb
  MATLAB Function : MATLAB Function  TreatAsAtomicUnit=on
  MatrixMultiply : Product  Multiplication=Matrix(*)
  MatrixMultiply1 : Product  Multiplication=Matrix(*)
  MatrixMultiply2 : Product  Multiplication=Matrix(*)
  Random Number : RandomNumber  Variance=sensors.eh.sigmaPhi^2  Seed=randi(1e5, 1, 1)  SampleTime=max([sensors.eh.Ts, sensors.st.Ts])
  Random Number1 : RandomNumber  Variance=sensors.eh.sigmaTheta^2  Seed=randi(1e5, 1, 1)  SampleTime=max([sensors.eh.Ts, sensors.st.Ts])
  Random Number2 : RandomNumber  Variance=sensors.eh.sigmaPsi^2  Seed=randi(1e5, 1, 1)  SampleTime=max([sensors.eh.Ts, sensors.st.Ts])
  Reshape : Reshape  OutputDimensionality=Column vector (2-D)
  Zero-Order Hold : ZeroOrderHold  SampleTime=max([sensors.eh.Ts, sensors.st.Ts])
  vEarth_b : Outport
  wires:
  Zero-Order Hold/1 -> MatrixMultiply1/2
  vEarth_n/1 -> MatrixMultiply2/2
  MATLAB Function/1(A_err) -> MatrixMultiply1/1
  Random Number2/1 -> MATLAB Function/3(psi)
  A_bn/1 -> MatrixMultiply2/1
  Random Number/1 -> MATLAB Function/1(phi)
  MatrixMultiply1/1 -> Reshape/1
  MatrixMultiply/1 -> Zero-Order Hold/1  "vEarth_s"
  Random Number1/1 -> MATLAB Function/2(theta)
  MatrixMultiply2/1 -> MatrixMultiply/2
  Constant/1 -> MatrixMultiply/1
  Reshape/1 -> vEarth_b/1

== system sadc_library_old/Sensors/Eclipse (S.T + E.H sensors)/Star tracker ==
  A_bn : Inport
  MATLAB Function : MATLAB Function  TreatAsAtomicUnit=on
  Memory : Memory  InitialCondition=sensors.st.vStars_n_init  InheritSampleTime=on
  Random Number : RandomNumber  Variance=sensors.st.sigmaPhi^2  Seed=randi(1e5,1,1)  SampleTime=max([sensors.eh.Ts, sensors.st.Ts])
  Random Number1 : RandomNumber  Variance=sensors.st.sigmaTheta^2  Seed=randi(1e5,1,1)  SampleTime=max([sensors.eh.Ts, sensors.st.Ts])
  Random Number2 : RandomNumber  Variance=sensors.st.sigmaPsi^2  Seed=randi(1e5,1,1)  SampleTime=max([sensors.eh.Ts, sensors.st.Ts])
  Zero-Order Hold : ZeroOrderHold  SampleTime=max([sensors.eh.Ts, sensors.st.Ts])
  sStars_b : Outport
  vStars_n : Outport  Port=2
  wires:
  Random Number1/1 -> MATLAB Function/3(theta)
  A_bn/1 -> Zero-Order Hold/1
  Random Number2/1 -> MATLAB Function/4(psi)
  Random Number/1 -> MATLAB Function/2(phi)
  Zero-Order Hold/1 -> MATLAB Function/1(A_bn)
  MATLAB Function/1(s_b) -> sStars_b/1
  MATLAB Function/2(v_n) -> Memory/1, vStars_n/1
  Memory/1 -> MATLAB Function/5(v_n_old)

== system sadc_library_old/Sensors/Sunlight (S.S + E.H sensors)/Earth-horizon sensor ==
  A_bn : Inport
  vEarth_n : Inport  Port=2
  Constant : Constant  Value=sensors.eh.A_sb
  MATLAB Function : MATLAB Function  TreatAsAtomicUnit=on
  MatrixMultiply : Product  Multiplication=Matrix(*)
  MatrixMultiply1 : Product  Multiplication=Matrix(*)
  MatrixMultiply2 : Product  Multiplication=Matrix(*)
  Random Number : RandomNumber  Variance=sensors.eh.sigmaPhi^2  Seed=randi(1e5, 1, 1)  SampleTime=max([sensors.ss.Ts, sensors.eh.Ts])
  Random Number1 : RandomNumber  Variance=sensors.eh.sigmaTheta^2  Seed=randi(1e5, 1, 1)  SampleTime=max([sensors.ss.Ts, sensors.eh.Ts])
  Random Number2 : RandomNumber  Variance=sensors.eh.sigmaPsi^2  Seed=randi(1e5, 1, 1)  SampleTime=max([sensors.ss.Ts, sensors.eh.Ts])
  Zero-Order Hold : ZeroOrderHold  SampleTime=max([sensors.ss.Ts, sensors.eh.Ts])
  vEarth_b : Outport
  wires:
  Constant/1 -> MatrixMultiply/1
  MatrixMultiply2/1 -> MatrixMultiply/2
  Random Number1/1 -> MATLAB Function/2(theta)
  MatrixMultiply/1 -> Zero-Order Hold/1  "vEarth_s"
  MatrixMultiply1/1 -> vEarth_b/1
  Random Number/1 -> MATLAB Function/1(phi)
  A_bn/1 -> MatrixMultiply2/1
  Random Number2/1 -> MATLAB Function/3(psi)
  MATLAB Function/1(A_err) -> MatrixMultiply1/1
  vEarth_n/1 -> MatrixMultiply2/2
  Zero-Order Hold/1 -> MatrixMultiply1/2

== system sadc_library_old/Sensors/Sunlight (S.S + E.H sensors)/Sun sensor ==
  A_bn : Inport
  vSun_n : Inport  Port=2
  Constant : Constant  Value=sensors.ss.A_sb
  If Action Subsystem : Subsystem  TreatAsAtomicUnit=on
  MatrixMultiply : Product  Multiplication=Matrix(*)
  MatrixMultiply2 : Product  Multiplication=Matrix(*)
  Measured Sun position : Subsystem  TreatAsAtomicUnit=on
  Merge : Merge
  Sensor FoV : Subsystem
  Zero-Order Hold : ZeroOrderHold  SampleTime=max([sensors.ss.Ts, sensors.eh.Ts])
  vSun_b : Outport
  wires:
  MatrixMultiply2/1 -> MatrixMultiply/2, Sensor FoV/2(vSun_b)
  MatrixMultiply/1 -> Zero-Order Hold/1  "vSun_s"
  A_bn/1 -> MatrixMultiply2/1
  vSun_n/1 -> MatrixMultiply2/2
  Constant/1 -> Sensor FoV/1(A_sb), MatrixMultiply/1
  If Action Subsystem/1(vSun_b) -> Merge/2
  Zero-Order Hold/1 -> Measured Sun position/1(vSun_s)
  Merge/1 -> vSun_b/1
  Sensor FoV/1(SunInFoV) -> If Action Subsystem/Enable, Measured Sun position/Enable
  Measured Sun position/1(vSun_b) -> Merge/1

== system sadc_library_old/Sensors1/Earth-horizon sensor/Determination of the sampling time ==
  NOR : Inport
  OR : Inport  Port=2
  Merge : Merge
  Merge1 : Merge
  Merge2 : Merge
  SS + EH : Subsystem  TreatAsAtomicUnit=on
  ST + EH : Subsystem  TreatAsAtomicUnit=on
  phi : Outport
  theta : Outport  Port=2
  psi : Outport  Port=3
  wires:
  ST + EH/3(psi) -> Merge2/1
  SS + EH/2(theta) -> Merge1/1
  ST + EH/1(phi) -> Merge/2
  SS + EH/3(psi) -> Merge2/2
  SS + EH/1(phi) -> Merge/1
  ST + EH/2(theta) -> Merge1/2
  Merge/1 -> phi/1
  Merge1/1 -> theta/1
  Merge2/1 -> psi/1
  NOR/1 -> SS + EH/Enable
  OR/1 -> ST + EH/Enable

== system sadc_library_old/Sensors/Sunlight (S.S + E.H sensors)/Sun sensor/If Action Subsystem ==
  Enable : EnablePort
  Constant : Constant  Value=[NaN; NaN; NaN]
  vSun_b : Outport
  wires:
  Constant/1 -> vSun_b/1

== system sadc_library_old/Sensors/Sunlight (S.S + E.H sensors)/Sun sensor/Measured Sun position ==
  vSun_s : Inport
  Enable : EnablePort
  MATLAB Function : MATLAB Function  TreatAsAtomicUnit=on
  MatrixMultiply1 : Product  Multiplication=Matrix(*)
  Random Number : RandomNumber  Variance=sensors.ss.sigmaPhi^2  Seed=randi(1e5, 1, 1)  SampleTime=max([sensors.ss.Ts, sensors.eh.Ts])
  Random Number1 : RandomNumber  Variance=sensors.ss.sigmaTheta^2  Seed=randi(1e5, 1, 1)  SampleTime=max([sensors.ss.Ts, sensors.eh.Ts])
  Random Number2 : RandomNumber  Variance=sensors.ss.sigmaPsi^2  Seed=randi(1e5, 1, 1)  SampleTime=max([sensors.ss.Ts, sensors.eh.Ts])
  vSun_b : Outport
  wires:
  vSun_s/1 -> MatrixMultiply1/2
  MATLAB Function/1(A_err) -> MatrixMultiply1/1
  MatrixMultiply1/1 -> vSun_b/1
  Random Number/1 -> MATLAB Function/1(phi)
  Random Number1/1 -> MATLAB Function/2(theta)
  Random Number2/1 -> MATLAB Function/3(psi)

== system sadc_library_old/Sensors/Sunlight (S.S + E.H sensors)/Sun sensor/Sensor FoV ==
  A_sb : Inport
  vSun_b : Inport  Port=2
  Acos : Trigonometry  Operator=acos
  Constant : Constant  Value=sensors.ss.FoV/2
  Dot Product : DotProduct  InputSameDT=on  OutDataTypeStr=Inherit: Inherit via internal rule
  Gain : Gain  Gain=sensors.ss.A_sb  Multiplication=Matrix(K*u) (u vector)
  Less Than : RelationalOperator  Operator=<=  OutDataTypeStr=boolean  RndMeth=Simplest
  Normalize Vector : vrlib/Utilities/Normalize Vector  maxzero=0
  Selector : Selector  NumberOfDimensions=2  InputPortWidth=3  IndexOptions=Index vector (dialog),Index vector (dialog)  Indices=[1 2 3],[1]  OutputSizes=1,1
  SunInFoV : Outport
  wires:
  Less Than/1 -> SunInFoV/1
  Constant/1 -> Less Than/2
  Acos/1 -> Less Than/1
  Dot Product/1 -> Acos/1
  vSun_b/1 -> Gain/1
  Normalize Vector/1 -> Dot Product/1
  Selector/1 -> Normalize Vector/1
  A_sb/1 -> Selector/1
  Gain/1 -> Dot Product/2

== system sadc_library_old/Sensors1/Earth-horizon sensor/Determination of the sampling time/SS + EH ==
  Enable : EnablePort
  Random Number : RandomNumber  Variance=sensors.eh.sigmaPhi^2  Seed=randi(1e5, 1, 1)  SampleTime=max([sensors.ss.Ts, sensors.eh.Ts])
  Random Number1 : RandomNumber  Variance=sensors.eh.sigmaTheta^2  Seed=randi(1e5, 1, 1)  SampleTime=max([sensors.ss.Ts, sensors.eh.Ts])
  Random Number2 : RandomNumber  Variance=sensors.eh.sigmaPsi^2  Seed=randi(1e5, 1, 1)  SampleTime=max([sensors.ss.Ts, sensors.eh.Ts])
  phi : Outport
  theta : Outport  Port=2
  psi : Outport  Port=3
  wires:
  Random Number1/1 -> theta/1
  Random Number2/1 -> psi/1
  Random Number/1 -> phi/1

== system sadc_library_old/Sensors1/Earth-horizon sensor/Determination of the sampling time/ST + EH ==
  Enable : EnablePort
  Random Number : RandomNumber  Variance=sensors.eh.sigmaPhi^2  Seed=randi(1e5, 1, 1)  SampleTime=max([sensors.st.Ts, sensors.eh.Ts])
  Random Number1 : RandomNumber  Variance=sensors.eh.sigmaTheta^2  Seed=randi(1e5, 1, 1)  SampleTime=max([sensors.st.Ts, sensors.eh.Ts])
  Random Number2 : RandomNumber  Variance=sensors.eh.sigmaPsi^2  Seed=randi(1e5, 1, 1)  SampleTime=max([sensors.st.Ts, sensors.eh.Ts])
  phi : Outport
  theta : Outport  Port=2
  psi : Outport  Port=3
  wires:
  Random Number1/1 -> theta/1
  Random Number2/1 -> psi/1
  Random Number/1 -> phi/1

== matlab function sadc_library_old/Environment/Gravity gradient torque/MATLAB Function2 ==
  data: i input; A_in output
function A_in = inertial_to_inclined(i)

A_in = [1, 0, 0;...
    0, cos(i), sin(i);...
    0, -sin(i), cos(i)];

end

== matlab function sadc_library_old/Sensors1/Earth-horizon sensor/MATLAB Function ==
  data: phi input; A_err output; theta input; psi input
function A_err = error_matrix(phi, theta, psi)

A_err = [cos(psi)*cos(theta), cos(psi)*sin(theta)*sin(phi) + sin(psi)*cos(phi),...
    -cos(psi)*sin(theta)*cos(phi) + sin(psi)*sin(phi);...
    -sin(psi)*cos(theta), -sin(psi)*sin(theta)*sin(phi) + cos(psi)*cos(phi),...
    sin(psi)*sin(theta)*cos(phi) + cos(psi)*sin(phi);...
    sin(theta), -cos(theta)*sin(phi), cos(theta)*cos(phi)];
            
end

== matlab function sadc_library_old/Environment/Drag/MATLAB Function1 ==
  data: rr input; vv input; A_bn input; rho input; Fdrag_b output; Mdrag output; surfaces parameter
function [Fdrag_b, Mdrag] = drag(rr, vv, A_bn, rho, surfaces)

we_vec = [0; 0; 7.2921150e-5];
cd = surfaces.cd;

r_surf_body = surfaces.body.r_surf;
r_surf_panels = surfaces.panels.r_surf;

n_body = surfaces.body.n;
n_panels = surfaces.panels.n;

A_body = surfaces.body.A;
A_panels = surfaces.panels.A;

nf_body = size(r_surf_body,1);
nf_panels = size(r_surf_panels,1);

vv_atm = cross(we_vec,rr*1e3); % [m/s]
vv_rel = vv*1e3 - vv_atm; % Relative velocity in inertial frame [m/s]
v_rel = norm(vv_rel);
vv_b = A_bn*vv_rel;
v_b = norm(vv_b);
v_vec = vv_b/v_b;

c = -1/2*rho*cd*v_rel^2.*v_vec;

Fdrag_b = zeros(3,1);
Mdrag = zeros(3,1);

for k = 1:nf_panels
        n_dot = dot(n_panels(k,:), v_vec);
    if n_dot > 0
        A_cross = A_panels(k)*n_dot;
        Fdrag_i = c*A_cross;
        Fdrag_b = Fdrag_b + Fdrag_i;
        Mdrag = Mdrag + cross(r_surf_panels(k,:)', Fdrag_b);
    end
end

for k = 1:nf_body
    n_dot = dot(n_body(k,:), v_vec);
    if n_dot > 0
        A_cross = A_body(k)*n_dot;
        Fdrag_i = c*A_cross;
        Fdrag_b = Fdrag_b + Fdrag_i;
        Mdrag = Mdrag + cross(r_surf_body(k,:)', Fdrag_b);
    end
end


% aggiungere questione su "ombra aerodinamica"
end

== matlab function sadc_library_old/Kinematics/DCM/MATLAB Function ==
  data: q input; Q output
function Q = skew_matrix(q)

q1 = q(1);
q2 = q(2);
q3 = q(3);

Q = [0, -q3, q2;...
    q3, 0, -q1;...
    -q2, q1, 0];

end

== matlab function sadc_library_old/Sensors1/Star tracker/MATLAB Function ==
  data: A_bn input; s_b output; phi input; theta input; psi input; v_n_old input; v_n output; sensors parameter
function [s_b, v_n] = starTracker(A_bn, phi, theta, psi, v_n_old, sensors)

A_sb = sensors.st.A_sb;
nStars = sensors.st.nStars;
FoV = sensors.st.FoV;

A_bs = A_sb';
A_ns = A_bn'*A_bs;

s_b = zeros(3,nStars); 
v_n = zeros(3,nStars);

El = zeros(nStars,1);
Az = zeros(nStars,1);

for k = 0:nStars-1
    
    s_b_old = A_bn*v_n_old(:,end-k);
    v_s_old = A_sb*s_b_old;
    
    El_old = asin(v_s_old(3));
    Az_old = acos(v_s_old(1)/cos(El_old));
    
    if v_s_old(2) <= 0
        El_old = 2*pi - El_old;
    end
    
    if abs(Az_old) > FoV(1)/2 || abs(El_old) > FoV(2)/2
        Az(end-k) = 0.2*FoV(1)*(-1 + 2*rand(1,1));
        El(end-k) = 0.2*FoV(2)*(-1 + 2*rand(1,1));
        v_s = [cos(El(end-k))*cos(Az(end-k));...
            cos(El(end-k))*sin(Az(end-k));...
            sin(El(end-k))];
        A_err = [cos(psi)*cos(theta), cos(psi)*sin(theta)*sin(phi) + sin(psi)*cos(phi),...
            -cos(psi)*sin(theta)*cos(phi) + sin(psi)*sin(phi);...
            -sin(psi)*cos(theta), -sin(psi)*sin(theta)*sin(phi) + cos(psi)*cos(phi),...
            sin(psi)*sin(theta)*cos(phi) + cos(psi)*sin(phi);...
            sin(theta), -cos(theta)*sin(phi), cos(theta)*cos(phi)];
    else
        A_err = eye(3);
        v_s = v_s_old;
    end
   
   s_s = A_err*v_s;
   s_b(1:3,end-k) = A_bs*s_s; 
   v_n(1:3,end-k) = A_ns*v_s;
   
end

end

== matlab function sadc_library_old/Sensors1/Sun sensor/MATLAB Function ==
  data: phi input; A_err output; theta input; psi input
function A_err = error_matrix(phi, theta, psi)

A_err = [cos(psi)*cos(theta), cos(psi)*sin(theta)*sin(phi) + sin(psi)*cos(phi),...
    -cos(psi)*sin(theta)*cos(phi) + sin(psi)*sin(phi);...
    -sin(psi)*cos(theta), -sin(psi)*sin(theta)*sin(phi) + cos(psi)*cos(phi),...
    sin(psi)*sin(theta)*cos(phi) + cos(psi)*sin(phi);...
    sin(theta), -cos(theta)*sin(phi), cos(theta)*cos(phi)];
            
end

== matlab function sadc_library_old/Sensors/Eclipse (S.T + E.H sensors)/Earth-horizon sensor/MATLAB Function ==
  data: phi input; A_err output; theta input; psi input
function A_err = error_matrix(phi, theta, psi)

A_err = [cos(psi)*cos(theta), cos(psi)*sin(theta)*sin(phi) + sin(psi)*cos(phi),...
    -cos(psi)*sin(theta)*cos(phi) + sin(psi)*sin(phi);...
    -sin(psi)*cos(theta), -sin(psi)*sin(theta)*sin(phi) + cos(psi)*cos(phi),...
    sin(psi)*sin(theta)*cos(phi) + cos(psi)*sin(phi);...
    sin(theta), -cos(theta)*sin(phi), cos(theta)*cos(phi)];
            
end

== matlab function sadc_library_old/Sensors/Eclipse (S.T + E.H sensors)/Star tracker/MATLAB Function ==
  data: A_bn input; s_b output; phi input; theta input; psi input; v_n_old input; v_n output; sensors parameter
function [s_b, v_n] = starTracker(A_bn, phi, theta, psi, v_n_old, sensors)

A_sb = sensors.st.A_sb;
nStars = sensors.st.nStars;
FoV = sensors.st.FoV;

A_bs = A_sb';
A_ns = A_bn'*A_bs;

s_b = zeros(3,nStars); 
v_n = zeros(3,nStars);

El = zeros(nStars,1);
Az = zeros(nStars,1);

for k = 0:nStars-1
    
    s_b_old = A_bn*v_n_old(:,end-k);
    v_s_old = A_sb*s_b_old;
    
    El_old = asin(v_s_old(3));
    Az_old = acos(v_s_old(1)/cos(El_old));
    
    if v_s_old(2) <= 0
        El_old = 2*pi - El_old;
    end
    
    if abs(Az_old) > FoV(1)/2 || abs(El_old) > FoV(2)/2
        Az(end-k) = 0.2*FoV(1)*(-1 + 2*rand(1,1));
        El(end-k) = 0.2*FoV(2)*(-1 + 2*rand(1,1));
        v_s = [cos(El(end-k))*cos(Az(end-k));...
            cos(El(end-k))*sin(Az(end-k));...
            sin(El(end-k))];
        A_err = [cos(psi)*cos(theta), cos(psi)*sin(theta)*sin(phi) + sin(psi)*cos(phi),...
            -cos(psi)*sin(theta)*cos(phi) + sin(psi)*sin(phi);...
            -sin(psi)*cos(theta), -sin(psi)*sin(theta)*sin(phi) + cos(psi)*cos(phi),...
            sin(psi)*sin(theta)*cos(phi) + cos(psi)*sin(phi);...
            sin(theta), -cos(theta)*sin(phi), cos(theta)*cos(phi)];
    else
        A_err = eye(3);
        v_s = v_s_old;
    end
   
   s_s = A_err*v_s;
   s_b(1:3,end-k) = A_bs*s_s; 
   v_n(1:3,end-k) = A_ns*v_s;
   
end

end

== matlab function sadc_library_old/Sensors/Sunlight (S.S + E.H sensors)/Earth-horizon sensor/MATLAB Function ==
  data: phi input; A_err output; theta input; psi input
function A_err = error_matrix(phi, theta, psi)

A_err = [cos(psi)*cos(theta), cos(psi)*sin(theta)*sin(phi) + sin(psi)*cos(phi),...
    -cos(psi)*sin(theta)*cos(phi) + sin(psi)*sin(phi);...
    -sin(psi)*cos(theta), -sin(psi)*sin(theta)*sin(phi) + cos(psi)*cos(phi),...
    sin(psi)*sin(theta)*cos(phi) + cos(psi)*sin(phi);...
    sin(theta), -cos(theta)*sin(phi), cos(theta)*cos(phi)];
            
end

== matlab function sadc_library_old/Environment/Magnetic torque/MATLAB Function1 ==
  data: m output; t input
function m = m_vector(t)

we = 7.2921150e-5;
m = [sind(11.5)*cos(we*t);...
    sind(11.5)*sin(we*t);...
    cosd(11.5)];

end

== matlab function sadc_library_old/Sensors/Sunlight (S.S + E.H sensors)/Sun sensor/Measured Sun position/MATLAB Function ==
  data: phi input; A_err output; theta input; psi input
function A_err = error_matrix(phi, theta, psi)

A_err = [cos(psi)*cos(theta), cos(psi)*sin(theta)*sin(phi) + sin(psi)*cos(phi),...
    -cos(psi)*sin(theta)*cos(phi) + sin(psi)*sin(phi);...
    -sin(psi)*cos(theta), -sin(psi)*sin(theta)*sin(phi) + cos(psi)*cos(phi),...
    sin(psi)*sin(theta)*cos(phi) + cos(psi)*sin(phi);...
    sin(theta), -cos(theta)*sin(phi), cos(theta)*cos(phi)];
            
end

== matlab function sadc_library_old/Environment/Magnetic torque/MATLAB Function ==
  data: m input; rr input; b_b output; A_bn input
function b_b = magnetic_dipole(m, rr, A_bn)

H0 = 3.009279157871533e-05;
Req = 6378.1*1e3;
r_norm = norm(rr);
r_vec = rr/norm(rr)*1e3;

b_n = Req^3*H0/(r_norm^3)*(3*dot(m,r_vec)*r_vec - m);

b_b = A_bn*b_n;

end

== matlab function sadc_library_old/Environment/Gravity gradient torque/MATLAB Function ==
  data: Mgg output; I input; c input
function Mgg = gravity_gradient(I, c)

G = 6.67408e-11;
me = 5.97237e24;
Req = 6371.8e3;

c1 = c(1);
c2 = c(2);
c3 = c(3);
Ix = I(1,1);
Iy = I(2,2);
Iz = I(3,3);

Mgg = 3*G*me/(Req^3)*[(Iz - Iy)*c2*c3;...
    (Ix - Iz)*c1*c3;...
    (Iy - Ix)*c1*c2];

end
